simulink model "readValues"  (R2022a)
settings: Solver=VariableStepAuto  StartTime=0.0  StopTime=10.0  RelTol=1e-3
values from neighbouring files (symbols this model uses):
  InvSetpoint = 0    [init.m]
  Setpoint = 0    [init.m]
settings Model: Creator=Usuario  LastModifiedBy=Usuario

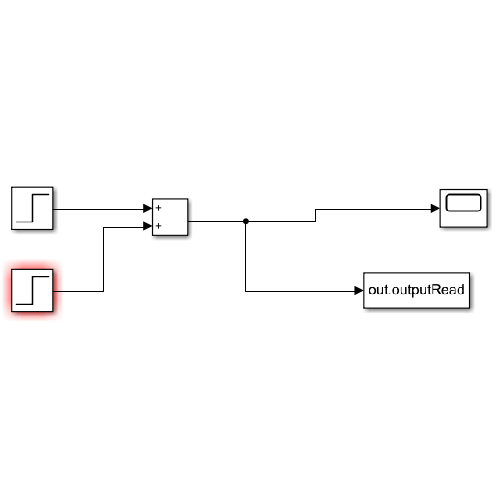
[thumbnail: Simulink's stored preview of the top-level diagram]
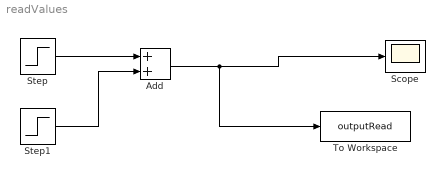
== system readValues ==
  Add : Sum
  Scope : Scope
  Step : Step  After=Setpoint  SampleTime=0
  Step1 : Step  Time=9  After=InvSetpoint  SampleTime=0
  To Workspace : ToWorkspace  VariableName=outputRead  SampleTime=-1
  wires:
  Step1/1 -> Add/2
  Step/1 -> Add/1
  Add/1 -> To Workspace/1, Scope/1
